simulink model "P5p5d"  (Simulink 9.0)
settings: Solver=ode45  StartTime=0.0  StopTime=400  RelTol=1e-3  EnableMultiTasking=on
undefined symbols (not defined in the file): K_pd, psi_r, T_d, T_f, T_s
libraries: simulink x2, simulink_extras x2
settings Model: SuppressorTable=22 serialization::archive 11 0 6 0 0 0 0 0  Creator=markh  LastModifiedBy=theodor
settings DataIOCC: LimitDataPoints=on  SignalLoggingSaveFormat=ModelDataLogs  SignalLoggingName=sigsOut
settings OptimizationCC: InitFltsAndDblsToZero=on
settings DebuggingCC: SaveWithParameterizedLinksMsg=none  SignalResolutionControl=TryResolveAllWithWarning  MultiTaskDSMMsg=warning  MultiTaskCondExecSysMsg=none  FcnCallInpInsideContextMsg=warning  StateNameClashWarn=warning
settings HardwareCC: TargetBitPerLong=64  TargetBitPerPointer=64  TargetBitPerSizeT=64  TargetBitPerPtrDiffT=64  TargetLongLongMode=on  TargetIntDivRoundTo=Zero  TargetEndianess=LittleEndian  TargetWordSize=64  TargetHWDeviceType=MATLAB Host  ProdEqTarget=off
settings GRTTargetCC: TargetFcnLib=ansi_tfl_tmw.mat  GeneratePreprocessorConditionals=Disable all  CombineOutputUpdateFcns=off  GRTInterface=on

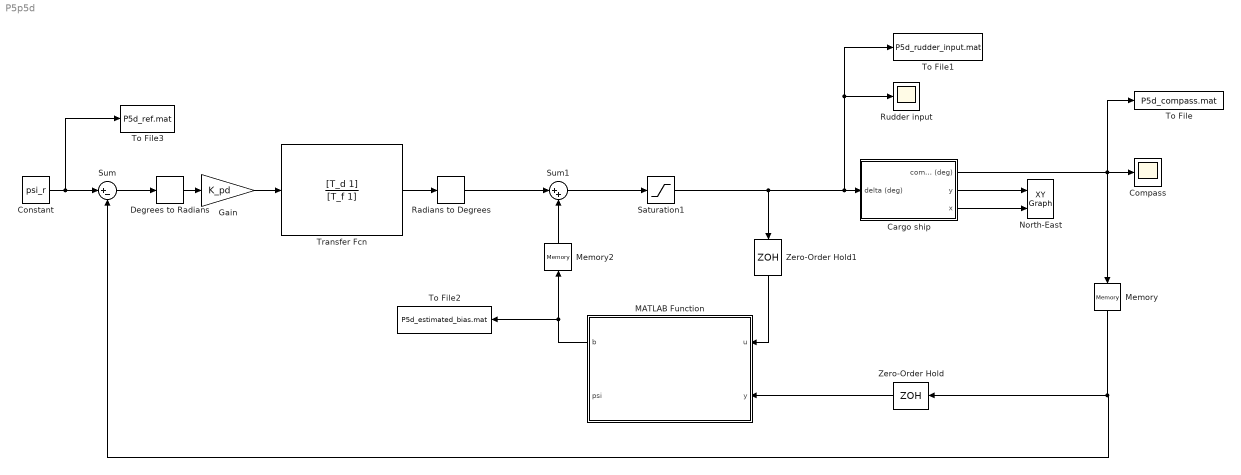
== system P5p5d ==
  Cargo ship : Subsystem  mask(Simple shipmodel for a cargo ship){noise=on, current=on, logic=off}
      mask prompts: noise "measurement noise"; logic "waves"
      mask help:
      | Measurement noise:
      | 	checked = noise on
      | 	unchecked = noise off
      |
      | Current:
      | 	checked = current on
      | 	unchecked = current off
      |
      | Waves:
      | 	checked = waves on
      | 	unchecked = waves off
      |
      | Author: Jørgen Spjøtvold, 9/10-2003
      | TTK 4115 Linear system theory.
      | Modified by Jostein Bakkeheim 26/10-2006
  "Compass " : Scope
  Constant : Constant  Value=psi_r
  Degrees to Radians : simulink_extras/Transformations/Degrees to Radians
  Gain : Gain  Gain=K_pd
  MATLAB Function : MATLAB Function  TreatAsAtomicUnit=on
  Memory : Memory
  Memory2 : Memory
  North-East : simulink/Sinks/XY Graph  xmin=-5000  xmax=5000  ymin=-5000  ymax=5000  st=-1
  Radians to Degrees : simulink_extras/Transformations/Radians to Degrees
  "Rudder input " : Scope
  Saturation1 : Saturate  UpperLimit=35  LowerLimit=-35
  Sum : Sum  Inputs=|+-
  Sum1 : Sum  Inputs=|++
  To File : ToFile  Filename=P5d_compass.mat  MatrixName=compass
  To File1 : ToFile  Filename=P5d_rudder_input.mat  MatrixName=rudder_input
  To File2 : ToFile  Filename=P5d_estimated_bias.mat  MatrixName=est_b
  To File3 : ToFile  Filename=P5d_ref.mat  MatrixName=ref
  Transfer Fcn : TransferFcn  Numerator=[T_d 1]  Denominator=[T_f 1]
  Zero-Order Hold : ZeroOrderHold  SampleTime=T_s
  Zero-Order Hold1 : ZeroOrderHold  SampleTime=T_s
  wires:
  Cargo ship/3(x) -> North-East/2
  Cargo ship/2(y) -> North-East/1
  Constant/1 -> To File3/1, Sum/1
  Sum/1 -> Degrees to Radians/1
  Gain/1 -> Transfer Fcn/1
  Degrees to Radians/1 -> Gain/1
  Cargo ship/1(compass (deg)) -> To File/1, "Compass "/1, Memory/1
  Transfer Fcn/1 -> Radians to Degrees/1
  Saturation1/1 -> "Rudder input "/1, To File1/1, Cargo ship/1(delta (deg)), Zero-Order Hold1/1
  Zero-Order Hold/1 -> MATLAB Function/2(y)
  MATLAB Function/1(b) -> To File2/1, Memory2/1
  Sum1/1 -> Saturation1/1
  Radians to Degrees/1 -> Sum1/1
  Memory/1 -> Sum/2, Zero-Order Hold/1
  Zero-Order Hold1/1 -> MATLAB Function/1(u)
  Memory2/1 -> Sum1/2

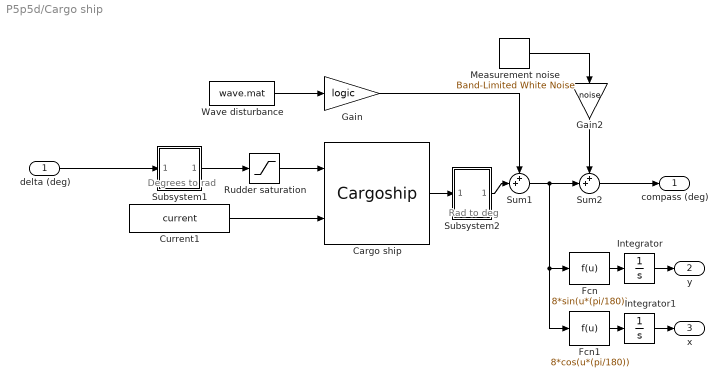
== system P5p5d/Cargo ship ==
  note: Degrees to rad
  note: Rad to deg
  delta (deg) : Inport
  Cargo ship : S-Function  FunctionName=Cargoship  SFunctionDeploymentMode=off  EnableBusSupport=off  mask(Cargo ship){}
      mask help:
      | S-function which simulates a cargo ship.
      |
      | Author: Jørgen Spjøtvold
      | 20.10-2003
      | Modified by Jostein Bakkeheim 27.10.2006
  Current1 : Constant  Value=current
  Fcn : Fcn  Expr=8*sin(u*(pi/180))
  Fcn1 : Fcn  Expr=8*cos(u*(pi/180))
  Gain : Gain  Gain=logic  SaturateOnIntegerOverflow=on  OutDataTypeStr=Inherit: Same as input  ParamDataTypeStr=Inherit: Same as input
  Gain2 : Gain  Gain=noise  SaturateOnIntegerOverflow=on  OutDataTypeStr=Inherit: Same as input  ParamDataTypeStr=Inherit: Same as input
  Integrator : Integrator
  Integrator1 : Integrator
  Measurement noise : simulink/Sources/Band-Limited White Noise  Cov=[0.001]  Ts=.5  seed=[23341]
  Rudder saturation : Saturate  UpperLimit=45*(pi/180)  LowerLimit=-45*(pi/180)
  Subsystem1 : Subsystem  mask(degrees to radians){}
      mask help: Converts degrees to radians
      mask Display: fprintf('D2R');
  Subsystem2 : Subsystem  mask(radians to degrees){}
      mask help: Converts radians to degrees
      mask Display: fprintf('R2D');
  Sum1 : Sum  Inputs=++|  SaturateOnIntegerOverflow=on
  Sum2 : Sum  Inputs=++|  SaturateOnIntegerOverflow=on
  Wave disturbance : FromFile  FileName=wave.mat  SampleTime=0
  compass (deg) : Outport
  y : Outport  Port=2
  x : Outport  Port=3
  wires:
  delta (deg)/1 -> Subsystem1/1(In1)
  Fcn/1 -> Integrator/1
  Integrator/1 -> y/1
  Fcn1/1 -> Integrator1/1
  Integrator1/1 -> x/1
  Wave disturbance/1 -> Gain/1
  Subsystem2/1(Out1) -> Sum1/2
  Gain/1 -> Sum1/1
  Sum1/1 -> Fcn/1, Fcn1/1, Sum2/2
  Cargo ship/1 -> Subsystem2/1(In1)
  Subsystem1/1(Out1) -> Rudder saturation/1
  Rudder saturation/1 -> Cargo ship/1
  Sum2/1 -> compass (deg)/1
  Measurement noise/1 -> Gain2/1
  Gain2/1 -> Sum2/1
  Current1/1 -> Cargo ship/2

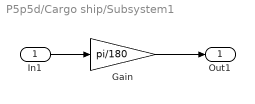
== system P5p5d/Cargo ship/Subsystem1 ==
  In1 : Inport
  Gain : Gain  Gain=pi/180  SaturateOnIntegerOverflow=on  OutDataTypeStr=Inherit: Same as input  ParamDataTypeStr=Inherit: Same as input
  Out1 : Outport
  wires:
  Gain/1 -> Out1/1
  In1/1 -> Gain/1

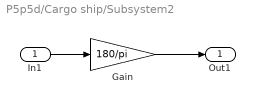
== system P5p5d/Cargo ship/Subsystem2 ==
  In1 : Inport
  Gain : Gain  Gain=180/pi  SaturateOnIntegerOverflow=on  OutDataTypeStr=Inherit: Same as input  ParamDataTypeStr=Inherit: Same as input
  Out1 : Outport
  wires:
  Gain/1 -> Out1/1
  In1/1 -> Gain/1

== matlab function MATLAB Function ==
  data: u input double; b output double; y input double; psi output double; sys parameter double
function [b, psi] = kalman_filter(u, y, sys)

persistent init_flag A B C E Q R Pm xm I

if (isempty(init_flag))
    init_flag = 1;
    
    [A, B, C, E, Q, R, Pm, xm, I] = deal(sys.A_d, sys.B_d, sys.C_d, sys.E_d, sys.Q, sys.R, sys.P_0m, sys.x_0m, sys.I);
            
end
% Kalman Gain
    L = (Pm*C')/(C*Pm*C'+R);
    
% Update Estimate
    x = xm + L*(y-C*xm);
 
% Update Error
    P = (I - L*C)*Pm*(I-L*C)' + L*R*L';
   
% Project ahead
    xm = A*x + B*u;
    Pm = A*P*A' + E*Q*E';
    
psi = x(3); b = x(5);

end
